simulink library "GFL_Lib"  (R2019b)
settings: Solver=VariableStepAuto  StartTime=0.0  StopTime=10.0  RelTol=1e-3
undefined symbols (not defined in the file or in its folder): Carm, Diff_CC_ki, Diff_CC_kp, fb, Ib2, Idcb, Ki_i, Ki_Wdiff_pu, Ki_Wtot_pu, Kp_i, Kp_Rvi_pu, Kp_Wdiff_pu, Kp_Wtot_pu, Lb, Lc_eq, Lc_pu, Lf_pu, Sb, Solver_Time_Step, Time_Step, Va0, Vb0, Vb1, Vb2, Vc0, Vdcb, Vm0, Vm0_d, Vm0_q, VSC01_id0, Vvsc0, wb, Zb
libraries: powerlib x90, Control_Lib x57, spsCurrentMeasurementLib x7, simulink x7, spsControlledCurrentSourceLib x6, $bdroot x5, Source_Lib x2, eeGeneralControl x2, powerlib_meascontrol x2, GFo_Lib x1
(part 3 of 5)

== system GFL_Lib/GFM_VC MMC/Bridge_Model ==
  vv_ref : Inport
  vdiff_ref : Inport  Port=2
  Bus1 : powerlib/Measurements/Three-Phase V-I Measurement  VoltageMeasurement=phase-to-ground  SetLabelV=off  LabelV=Vabc  Vpu=off  VpuLL=off  CurrentMeasurement=no  SetLabelI=off  LabelI=Iabc  Ipu=off  Pbase=100e6  Vbase=500e3  OutputType=Complex  PhasorSimulation=off  PSBequivalent=0
  Current Measurement : spsCurrentMeasurementLib/Current Measurement  PhasorSimulation=off  OutputType=Complex  PSBequivalent=0
  Decoupling voltage : Subsystem
  MMC Average Model : Subsystem
  Memory1 : Memory  InitialCondition=Udcn
  Modulation Index Generation : Subsystem
  Mux : Mux  Inputs=2
  NOT1 : Logic  Operator=NOT  IconShape=distinctive  AllPortsSameDT=off  OutDataTypeStr=boolean
  Step : Step  Time=Output_Delay  SampleTime=0
  Three-Phase Breaker1 : powerlib/Elements/Three-Phase Breaker  InitialState=closed  SwitchA=on  SwitchB=on  SwitchC=on  SwitchTimes="[4/60  10/60]"  External=on  BreakerResistance=1e-5*Zb  SnubberResistance=1e6  SnubberCapacitance=inf  Measurements=None
  Three-Phase Breaker2 : powerlib/Elements/Three-Phase Breaker  InitialState=open  SwitchA=on  SwitchB=on  SwitchC=on  SwitchTimes="[4/60  10/60]"  External=on  BreakerResistance=1e-5*Zb  SnubberResistance=1e6  SnubberCapacitance=inf  Measurements=None
  Three-Phase Source : powerlib/Electrical Sources/Three-Phase Source  InternalConnection=Yg  VoltagePhases=off  Voltage=Vm0*Un1  PhaseAngle=Theta_Vm0  Voltage_phases=[25e3 25e3 25e3]/sqrt(3)  PhaseAngles_phases=[0 -120 +120]  Frequency=fb  NonIdealSource=on  SpecifyImpedance=off  Resistance=Rarm_pu/2*Zb  Inductance=Larm_pu/2*Lb  ShortCircuitLevel=100e6  BaseVoltage=Un1  XRratio=7  BusType=swing  Pref=0.3  Qref=0  Prefabc=[10e3, 10e3, 10e3]  Qrefabc=[0, 0, 0]  Qmin=-Inf  Qmax=Inf
  Voltage Measurement : powerlib/Measurements/Voltage Measurement  PhasorSimulation=off  OutputType=Complex  PSBequivalent=0
  PhA : PMIOPort  Side=Right
  PhB : PMIOPort  Port=2  Side=Right
  PhC : PMIOPort  Port=3  Side=Right
  Vdc+ : PMIOPort  Port=4  Side=Left
  Vdc- : PMIOPort  Port=5  Side=Left
  m_dc : Outport
  m : Outport  Port=2
  vv : Outport  Port=3
  wires:
  NOT1/1 -> Three-Phase Breaker1/1
  Step/1 -> Three-Phase Breaker2/1, NOT1/1
  vv_ref/1 -> Decoupling voltage/1(Vv_ref)
  vdiff_ref/1 -> Decoupling voltage/2(Vdiff_ref)
  Decoupling voltage/1(Vmu_ref) -> Modulation Index Generation/1(vmu_ref)
  Decoupling voltage/2(Vml_ref) -> Modulation Index Generation/2(vml_ref)
  MMC Average Model/1(m) -> m/1
  Voltage Measurement/1 -> Memory1/1  "Vdc"
  Current Measurement/1 -> Mux/2  "Idc"
  Mux/1 -> m_dc/1
  Modulation Index Generation/1(mul) -> MMC Average Model/1(mul)
  Bus1/1 -> vv/1
  Memory1/1 -> Mux/1
  connections:
  Three-Phase Breaker1/LConn1 -- Bus1/LConn1 -- Three-Phase Breaker2/LConn1
  Three-Phase Breaker1/LConn2 -- Bus1/LConn2 -- Three-Phase Breaker2/LConn2
  Three-Phase Breaker1/LConn3 -- Bus1/LConn3 -- Three-Phase Breaker2/LConn3
  MMC Average Model/LConn1 -- Three-Phase Breaker2/RConn1
  MMC Average Model/LConn2 -- Three-Phase Breaker2/RConn2
  MMC Average Model/LConn3 -- Three-Phase Breaker2/RConn3
  Three-Phase Source/RConn1 -- Three-Phase Breaker1/RConn1
  Three-Phase Source/RConn2 -- Three-Phase Breaker1/RConn2
  Three-Phase Source/RConn3 -- Three-Phase Breaker1/RConn3
  MMC Average Model/RConn1 -- Current Measurement/RConn1 -- Voltage Measurement/LConn1
  MMC Average Model/RConn2 -- Voltage Measurement/LConn2 -- Vdc-/RConn1
  Current Measurement/LConn1 -- Vdc+/RConn1
  PhB/RConn1 -- Bus1/RConn2
  PhC/RConn1 -- Bus1/RConn3
  PhA/RConn1 -- Bus1/RConn1

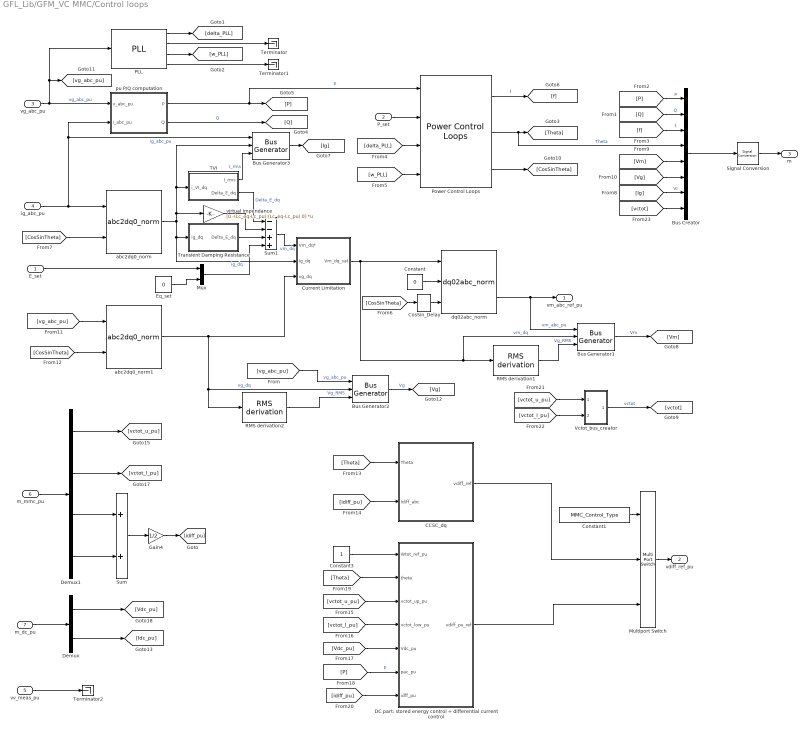
== system GFL_Lib/GFM_VC MMC/Control loops ==
  E_set : Inport
  P_set : Inport  Port=2
  vg_abc_pu : Inport  Port=3
  ig_abc_pu : Inport  Port=4
  vv_meas_pu : Inport  Port=5
  m_mmc_pu : Inport  Port=6
  m_dc_pu : Inport  Port=7
  " pu P/Q computation" : Subsystem  DialogController=POWERSYS.PowerSysDialog
  Bus Creator : BusCreator  Inputs=8
  Bus Generator1 : Control_Lib/Bus Generator  Gpu=Vb1
      settings: SourceProductName=VSC4SPS
  Bus Generator2 : Control_Lib/Bus Generator  Gpu=Vb1
      settings: SourceProductName=VSC4SPS
  Bus Generator3 : Control_Lib/Bus Generator  Gpu=Vb1
      settings: SourceProductName=VSC4SPS
  CCSC_dq : Subsystem
  Constant : Constant  Value=0
  Constant1 : Constant  Value=MMC_Control_Type
  Constant3 : Constant
  CosSin_Delay : Control_Lib/CosSin_Delay  dTheta=wb*Output_Delay
      settings: SourceProductName=VSC4SPS
  Current Limitation : Subsystem
  DC part: stored energy control + differential current control : Subsystem
  Demux : Demux  Outputs=2
  Demux1 : Demux  Outputs=[3 3 3 3]
  Eq_set : Constant  Value=0
  Gain4 : Gain  Gain=1/2
  Multiport Switch : MultiPortSwitch  Inputs=2
  Mux : Mux  Inputs=2
  PLL : Control_Lib/PLL  fb=fb  wn_PLL=wn_PLL  zeta_PLL=zeta_PLL  Theta0=Theta0
      settings: SourceProductName=VSC4SPS
  Power Control Loops : Control_Lib/Power Control Loops  Theta0_VSC=Theta_Vvsc0
      settings: SourceProductName=VSC4SPS
  RMS derivation1 : Control_Lib/RMS derivation  SystemSampleTime=-1  Latency=0  AutoFrameSizeCalculation=off
      settings: SourceProductName=VSC4SPS
  RMS derivation2 : Control_Lib/RMS derivation  SystemSampleTime=-1  Latency=0  AutoFrameSizeCalculation=off
      settings: SourceProductName=VSC4SPS
  Signal Conversion : SignalConversion  OverrideOpt=off
  Sum : Sum
  Sum1 : Sum  Inputs=--++
  TVI : Subsystem
  Terminator : Terminator
  Terminator1 : Terminator
  Terminator2 : Terminator
  Transient Damping Resistance : Subsystem
  Vctot_bus_creator : Subsystem
  abc2dq0_norm : Control_Lib/abc2dq0_norm  referenceAxisMode=Reference axis at 90 degrees behind phase_a  baseUpdateGain=1/sqrt(3)
      settings: SourceProductName=VSC4SPS
  abc2dq0_norm1 : Control_Lib/abc2dq0_norm  referenceAxisMode=Reference axis at 90 degrees behind phase_a  baseUpdateGain=1/sqrt(3)
      settings: SourceProductName=VSC4SPS
  dq02abc_norm : Control_Lib/dq02abc_norm  referenceAxisMode=Reference axis at 90 degrees behind phase_a  baseUpdateGain=sqrt(3)
      settings: SourceProductName=VSC4SPS
  virtual impendance : Gain  Gain=[0 -(Lc_eq-Lc_pu);(Lc_eq-Lc_pu) 0]  Multiplication=Matrix(K*u)
  vm_abc_ref_pu : Outport  VectorParamsAs1DForOutWhenUnconnected=off
  vdiff_ref_pu : Outport  Port=2
  m : Outport  Port=3  VectorParamsAs1DForOutWhenUnconnected=off
  wires:
  vv_meas_pu/1 -> Terminator2/1
  [vctot] -> Bus Creator/8
  [vctot_l_pu] -> Vctot_bus_creator/2(In2)
  Vctot_bus_creator/1(Out1) -> [vctot]  "vctot"
  [vctot_u_pu] -> Vctot_bus_creator/1(In1)
  Multiport Switch/1 -> vdiff_ref_pu/1
  PLL/4 -> Terminator1/1
  PLL/2 -> Terminator/1
  PLL/1 -> [delta_PLL]
  Constant/1 -> dq02abc_norm/2
  Power Control Loops/3 -> [CosSinTheta]
  PLL/3 -> [w_PLL]
  [Vg] -> Bus Creator/6
  Bus Creator/1 -> Signal Conversion/1
  [Ig] -> Bus Creator/7  "VI"
  [Vm] -> Bus Creator/5
  Eq_set/1 -> Mux/2
  Mux/1 -> Sum1/4
  TVI/1(I_rms) -> Bus Generator3/3  "I_rms"
  Transient Damping Resistance/1("Delta_E_dq ") -> Sum1/3
  TVI/2(Delta_E_dq) -> Sum1/1  "Delta_E_dq"
  [CosSinTheta] -> abc2dq0_norm/2
  [CosSinTheta] -> CosSin_Delay/1
  Power Control Loops/2 -> Bus Creator/4, [Theta]  "Theta"
  abc2dq0_norm/2 -> Transient Damping Resistance/1(ig_dq), Current Limitation/2(Ig_dq), Bus Generator3/2, TVI/1(i_VI_dq), virtual impendance/1  "ig_dq"
  ig_abc_pu/1 -> abc2dq0_norm/1, Bus Generator3/1, " pu P/Q computation"/2(i_abc_pu)  "ig_abc_pu"
  " pu P/Q computation"/1(P) -> Power Control Loops/1, [P]  "P"
  vg_abc_pu/1 -> PLL/1, [vg_abc_pu], " pu P/Q computation"/1(v_abc_pu)  "vg_abc_pu"
  Power Control Loops/1 -> [f]  "f"
  P_set/1 -> Power Control Loops/2
  [delta_PLL] -> Power Control Loops/3
  Current Limitation/1(Vm_dq_sat) -> Bus Generator1/2, RMS derivation1/1, dq02abc_norm/1  "vm_dq"
  " pu P/Q computation"/2(Q) -> [Q]  "Q"
  E_set/1 -> Mux/1
  dq02abc_norm/2 -> Bus Generator1/1, vm_abc_ref_pu/1  "vm_abc_pu"
  [f] -> Bus Creator/3  "f"
  [Q] -> Bus Creator/2  "Q"
  [P] -> Bus Creator/1  "P"
  Signal Conversion/1 -> m/1
  Sum1/1 -> Current Limitation/1(Vm_dq*)  "vm_dq"
  [vg_abc_pu] -> abc2dq0_norm1/1
  [CosSinTheta] -> abc2dq0_norm1/2
  Demux1/2 -> [vctot_l_pu]
  Demux1/1 -> [vctot_u_pu]
  m_mmc_pu/1 -> Demux1/1
  Demux/2 -> [Idc_pu]
  Demux/1 -> [Vdc_pu]
  m_dc_pu/1 -> Demux/1
  Gain4/1 -> [idiff_pu]
  Sum/1 -> Gain4/1
  Demux1/3 -> Sum/1
  Demux1/4 -> Sum/2
  [vctot_u_pu] -> DC part: stored energy control + differential current control/3(vctot_up_pu)
  [vctot_l_pu] -> DC part: stored energy control + differential current control/4(vctot_low_pu)
  [Vdc_pu] -> DC part: stored energy control + differential current control/5(Vdc_pu)
  [P] -> DC part: stored energy control + differential current control/6(pac_pu)  "P"
  Constant3/1 -> DC part: stored energy control + differential current control/1(Wtot_ref_pu)
  [Theta] -> DC part: stored energy control + differential current control/2(theta)
  [idiff_pu] -> DC part: stored energy control + differential current control/7(idff_pu)
  [w_PLL] -> Power Control Loops/4
  CosSin_Delay/1 -> dq02abc_norm/3
  [Theta] -> CCSC_dq/1(Theta)
  CCSC_dq/1(vdiff_ref) -> Multiport Switch/2
  [idiff_pu] -> CCSC_dq/2(Idiff_abc)
  virtual impendance/1 -> Sum1/2
  DC part: stored energy control + differential current control/1(vdiff_pu_ref) -> Multiport Switch/3
  Constant1/1 -> Multiport Switch/1
  Bus Generator1/1 -> [Vm]  "Vm"
  RMS derivation1/1 -> Bus Generator1/3  "Vg_RMS"
  RMS derivation2/1 -> Bus Generator2/3  "Vg_RMS"
  Bus Generator2/1 -> [Vg]  "Vg"
  [vg_abc_pu] -> Bus Generator2/1  "vg_abc_pu"
  abc2dq0_norm1/2 -> RMS derivation2/1, Bus Generator2/2, Current Limitation/3(vg_dq)  "vg_dq"
  Bus Generator3/1 -> [Ig]

== system GFL_Lib/GFM_VC MMC/Normalization_dc ==
  m_dc : Inport
  Demux : Demux  Outputs=2
  Gain11 : Gain  Gain=1/Vdcb
  Gain12 : Gain  Gain=1/Idcb
  Mux : Mux  Inputs=2
  m_dc_pu : Outport
  wires:
  Mux/1 -> m_dc_pu/1
  Demux/2 -> Gain12/1
  Gain12/1 -> Mux/2  "Idc_pu"
  Gain11/1 -> Mux/1  "Vdc_pu"
  Demux/1 -> Gain11/1
  m_dc/1 -> Demux/1

== system GFL_Lib/GFM_VC MMC/Normalizaton ==
  m_mmc : Inport
  Demux : Demux  Outputs=[3 3 3 3]
  Gain : Gain  Gain=1/Idcb
  Gain3 : Gain  Gain=1/Idcb
  Gain6 : Gain  Gain=1/Vdcb
  Gain8 : Gain  Gain=1/Vdcb
  Mux : Mux
  m_mmc_pu : Outport
  wires:
  m_mmc/1 -> Demux/1
  Mux/1 -> m_mmc_pu/1
  Demux/3 -> Gain/1
  Gain/1 -> Mux/3  "i_arm_u_pu"
  Demux/4 -> Gain3/1
  Gain3/1 -> Mux/4  "i_arm_l_pu"
  Demux/2 -> Gain8/1
  Gain6/1 -> Mux/1  "vctot_u_pu"
  Demux/1 -> Gain6/1
  Gain8/1 -> Mux/2  "vctot_l_pu"

== system GFL_Lib/Mean Model 2-Level L-filter with DC Link/Bridge_Model ==
  Uref : Inport
  Constant : Constant
  Memory1 : Memory
  NOT1 : Logic  Operator=NOT  IconShape=distinctive  AllPortsSameDT=off  OutDataTypeStr=boolean
  Saturation : Saturate  UpperLimit=1  LowerLimit=-1
  Terminator : Terminator
  Three-Phase Breaker2 : powerlib/Elements/Three-Phase Breaker  InitialState=open  SwitchA=on  SwitchB=on  SwitchC=on  SwitchTimes="[4/60  10/60]"  External=on  BreakerResistance=1e-5*Zb  SnubberResistance=1e6  SnubberCapacitance=inf  Measurements=None
  Three-Phase Breaker3 : powerlib/Elements/Three-Phase Breaker  InitialState=closed  SwitchA=on  SwitchB=on  SwitchC=on  SwitchTimes="[4/60  10/60]"  External=on  BreakerResistance=1e-5*Zb  SnubberResistance=1e6  SnubberCapacitance=inf  Measurements=None
  Three-Phase Source : powerlib/Electrical Sources/Three-Phase Source  InternalConnection=Yg  VoltagePhases=off  Voltage=Vvsc0*Un1  PhaseAngle=Theta_vsc0  Voltage_phases=[25e3 25e3 25e3]/sqrt(3)  PhaseAngles_phases=[0 -120 +120]  Frequency=fb  NonIdealSource=off  SpecifyImpedance=off  Resistance=0  Inductance=0  ShortCircuitLevel=100e6  BaseVoltage=VSC01_Un1  XRratio=7  BusType=swing  Pref=0.3  Qref=0  Prefabc=[10e3, 10e3, 10e3]  Qrefabc=[0, 0, 0]  Qmin=-Inf  Qmax=Inf
  Universal Bridge : powerlib/Power Electronics/Universal Bridge  Arms=3  SnubberResistance=1e5  SnubberCapacitance=inf  Device=Average-model based VSC  Ron=1e-3  Lon=0  ForwardVoltages="[  0  0  ]"  ForwardVoltage=0  GTOparameters=[ 10e-6 , 20e-6 ]  IGBTparameters=[ 1e-6 , 2e-6 ]  Measurements=None  Measurements_2=None  converterType=Rectifier
  Vdc : powerlib/Measurements/Voltage Measurement  PhasorSimulation=off  OutputType=Complex  PSBequivalent=0
  mp3 : Gain  Gain=2/Udcn
  PhA : PMIOPort  Side=Right
  PhB : PMIOPort  Port=2  Side=Right
  PhC : PMIOPort  Port=3  Side=Right
  Vdc+ : PMIOPort  Port=4  Side=Left
  Vdc- : PMIOPort  Port=5  Side=Left
  wires:
  Vdc/1 -> Terminator/1
  Uref/1 -> mp3/1
  mp3/1 -> Saturation/1
  Constant/1 -> Memory1/1
  NOT1/1 -> Three-Phase Breaker3/1
  Saturation/1 -> Universal Bridge/1
  Memory1/1 -> Three-Phase Breaker2/1, NOT1/1
  connections:
  Vdc-/RConn1 -- Universal Bridge/RConn2 -- Vdc/LConn2
  Vdc+/RConn1 -- Universal Bridge/RConn1 -- Vdc/LConn1
  PhC/RConn1 -- Three-Phase Breaker3/LConn3 -- Three-Phase Breaker2/LConn3
  PhB/RConn1 -- Three-Phase Breaker3/LConn2 -- Three-Phase Breaker2/LConn2
  PhA/RConn1 -- Three-Phase Breaker3/LConn1 -- Three-Phase Breaker2/LConn1
  Three-Phase Breaker2/RConn3 -- Universal Bridge/LConn3
  Three-Phase Breaker2/RConn2 -- Universal Bridge/LConn2
  Three-Phase Breaker2/RConn1 -- Universal Bridge/LConn1
  Three-Phase Breaker3/RConn1 -- Three-Phase Source/RConn1
  Three-Phase Breaker3/RConn2 -- Three-Phase Source/RConn2
  Three-Phase Breaker3/RConn3 -- Three-Phase Source/RConn3

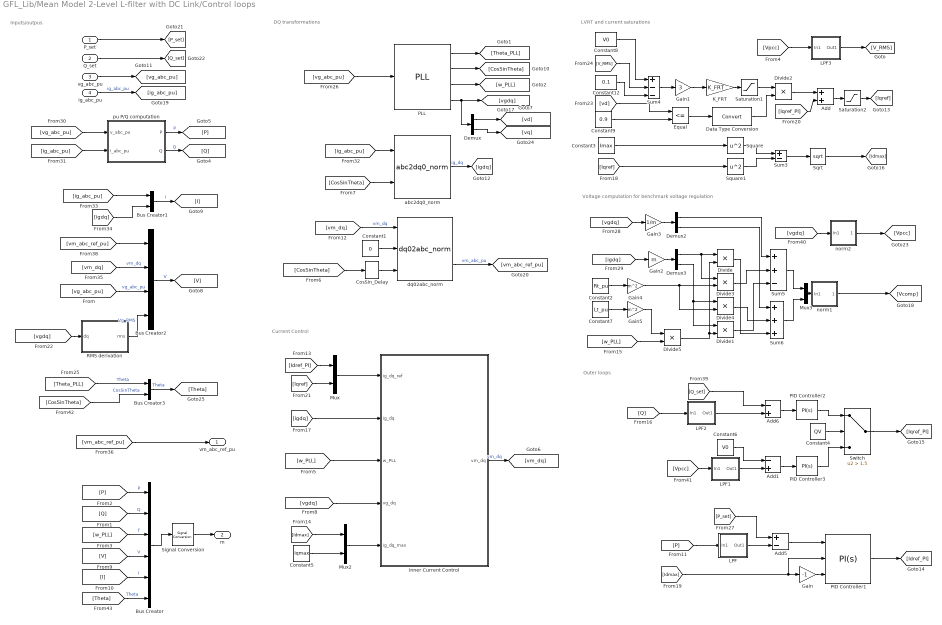
== system GFL_Lib/Mean Model 2-Level L-filter with DC Link/Control loops ==
  note: Voltage computation for benchmark voltage regulation
  note: LVRT and current saturations
  note: Outer loops
  note: Current Control
  note: DQ transformations
  note: Inputs/outpus
  P_set : Inport
  Q_set : Inport  Port=2
  vg_abc_pu : Inport  Port=3
  ig_abc_pu : Inport  Port=4
  " pu P/Q computation" : Subsystem  DialogController=POWERSYS.PowerSysDialog
  Add : Sum
  Add1 : Sum  Inputs=-+
  Add5 : Sum  Inputs=+-
  Add6 : Sum  Inputs=-+
  Bus Creator : BusCreator  Inputs=6
  Bus Creator1 : BusCreator  Inputs=2
  Bus Creator2 : BusCreator  Inputs=4
  Bus Creator3 : BusCreator  Inputs=2
  Constant1 : Constant  Value=0
  Constant12 : Constant  Value=0.1
  Constant2 : Constant  Value=Rt_pu
  Constant3 : Constant  Value=Imax
  Constant4 : Constant  Value=QV
  Constant5 : Constant  Value=Iqmax
  Constant6 : Constant  Value=V0
  Constant7 : Constant  Value=Lt_pu
  Constant8 : Constant  Value=V0
  Constant9 : Constant  Value=0.9
  CosSin_Delay : Control_Lib/CosSin_Delay  dTheta=wb*Solver_Time_Step
      settings: SourceProductName=VSC4SPS
  Data Type Conversion : DataTypeConversion
  Demux : Demux  Outputs=[1 1]
  Demux2 : Demux  Outputs=2
  Demux3 : Demux  Outputs=2
  Divide{,1..5} (6 alike) : Product  Inputs=**
  Equal : RelationalOperator  Operator=<=  OutDataTypeStr=boolean  RndMeth=Simplest
  Gain : Gain  Gain=-1
  Gain1 : Gain  Gain=3
  Gain2 : Gain  Gain=m
  Gain3 : Gain  Gain=1/m
  Gain4 : Gain  Gain=m^2
  Gain5 : Gain  Gain=m^2
  Inner Current Control : Subsystem
  K_FRT : Gain  Gain=K_FRT
  LPF : Subsystem
  LPF1 : Subsystem
  LPF2 : Subsystem
  LPF3 : Subsystem
  Mux : Mux  Inputs=2
  Mux2 : Mux  Inputs=2
  Mux3 : Mux  Inputs=2
  PID Controller1 : simulink/Continuous/PID Controller  Controller=PI  Form=Parallel  TimeDomain=Continuous-time  SampleTime=-1  IntegratorMethod=Forward Euler  FilterMethod=Forward Euler  ControllerParametersSource=internal  P=w_P/w_LPF  I=w_P  D=0  UseFilter=on  N=100  TunerSelectOption=Transfer Function Based (PID Tuner App)  InitialConditionSource=internal  InitialConditionForIntegrator=P0/V0  InitialConditionForFilter=0  DifferentiatorICPrevScaledInput=0  ExternalReset=none  TrackingMode=off  Kt=1  LimitOutput=on  UpperSaturationLimit=inf  LowerSaturationLimit=-inf  LinearizeAsGain=on  AntiWindupMode=clamping  Kb=1  POutMin=[]  POutMax=[]  IOutMin=[]  IOutMax=[]  DOutMin=[]  DOutMax=[]  NOutMin=[]  NOutMax=[]  SumOutMin=[]  SumOutMax=[]  SaturationOutMin=[]  SaturationOutMax=[]  PParamMin=[]  PParamMax=[]  IParamMin=[]  IParamMax=[]  DParamMin=[]  DParamMax=[]  NParamMin=[]  NParamMax=[]  KbParamMin=[]  KbParamMax=[]  KtParamMin=[]  KtParamMax=[]  KbOutMin=[]  KbOutMax=[]  KtOutMin=[]  KtOutMax=[]  IntegratorOutMin=[]  IntegratorOutMax=[]  FilterOutMin=[]  FilterOutMax=[]  SumI1OutMin=[]  SumI1OutMax=[]  SumI2OutMin=[]  SumI2OutMax=[]  SumI3OutMin=[]  SumI3OutMax=[]  SumI4OutMin=[]  SumI4OutMax=[]  SumDOutMin=[]  SumDOutMax=[]  DifferentiatorOutMin=[]  DifferentiatorOutMax=[]  FilterDiffOutCoefMin=[]  FilterDiffOutCoefMax=[]  ReciprocalOutMin=[]  ReciprocalOutMax=[]  SumDenOutMin=[]  SumDenOutMax=[]  SumNumOutMin=[]  SumNumOutMax=[]  DivideOutMin=[]  DivideOutMax=[]  IntegratorContinuousStateAttributes=''  IntegratorStateMustResolveToSignalObject=off  IntegratorRTWStateStorageClass=Auto  FilterContinuousStateAttributes=''  FilterStateMustResolveToSignalObject=off  FilterRTWStateStorageClass=Auto  ParallelPVariant=InternalParameters  IdealPVariant=Disabled  IVariant=InternalParameters  DVariant=Disabled  IntegratorVariant=Continuous  SatVariant=External  AWVariant=ContClampingParallel  PCopyVariant=Disabled  TRVariant=Disabled  FdbkBlocksVariant=Forward  IdealPFdbkVariant=Disabled  SatFdbkVariant=Disabled  DerivativeFilterVariant=Disabled  NVariant=Disabled  NCopyVariant=Disabled_SignalSpec  FilterICVariant=Disabled  IntegratorICVariant=InternalICs  ExternalResetVariant=Disabled  TRSumVariant=Passthrough  SumFdbkVariant=Disabled  SumVariant=Sum_PI
  PID Controller2 : simulink/Continuous/PID Controller  Controller=PI  Form=Parallel  TimeDomain=Continuous-time  SampleTime=-1  IntegratorMethod=Forward Euler  FilterMethod=Forward Euler  ControllerParametersSource=internal  P=w_P/w_LPF  I=w_P  D=0  UseFilter=on  N=100  TunerSelectOption=Transfer Function Based (PID Tuner App)  InitialConditionSource=internal  InitialConditionForIntegrator=-Q0/V0  InitialConditionForFilter=0  DifferentiatorICPrevScaledInput=0  ExternalReset=none  TrackingMode=off  Kt=1  LimitOutput=on  UpperSaturationLimit=Iqmax  LowerSaturationLimit=-Iqmax  LinearizeAsGain=on  AntiWindupMode=clamping  Kb=1  POutMin=[]  POutMax=[]  IOutMin=[]  IOutMax=[]  DOutMin=[]  DOutMax=[]  NOutMin=[]  NOutMax=[]  SumOutMin=[]  SumOutMax=[]  SaturationOutMin=[]  SaturationOutMax=[]  PParamMin=[]  PParamMax=[]  IParamMin=[]  IParamMax=[]  DParamMin=[]  DParamMax=[]  NParamMin=[]  NParamMax=[]  KbParamMin=[]  KbParamMax=[]  KtParamMin=[]  KtParamMax=[]  KbOutMin=[]  KbOutMax=[]  KtOutMin=[]  KtOutMax=[]  IntegratorOutMin=[]  IntegratorOutMax=[]  FilterOutMin=[]  FilterOutMax=[]  SumI1OutMin=[]  SumI1OutMax=[]  SumI2OutMin=[]  SumI2OutMax=[]  SumI3OutMin=[]  SumI3OutMax=[]  SumI4OutMin=[]  SumI4OutMax=[]  SumDOutMin=[]  SumDOutMax=[]  DifferentiatorOutMin=[]  DifferentiatorOutMax=[]  FilterDiffOutCoefMin=[]  FilterDiffOutCoefMax=[]  ReciprocalOutMin=[]  ReciprocalOutMax=[]  SumDenOutMin=[]  SumDenOutMax=[]  SumNumOutMin=[]  SumNumOutMax=[]  DivideOutMin=[]  DivideOutMax=[]  IntegratorContinuousStateAttributes=''  IntegratorStateMustResolveToSignalObject=off  IntegratorRTWStateStorageClass=Auto  FilterContinuousStateAttributes=''  FilterStateMustResolveToSignalObject=off  FilterRTWStateStorageClass=Auto  ParallelPVariant=InternalParameters  IdealPVariant=Disabled  IVariant=InternalParameters  DVariant=Disabled  IntegratorVariant=Continuous  SatVariant=Enabled  AWVariant=ContClampingParallel  PCopyVariant=Disabled  TRVariant=Disabled  FdbkBlocksVariant=Forward  IdealPFdbkVariant=Disabled  SatFdbkVariant=Disabled  DerivativeFilterVariant=Disabled  NVariant=Disabled  NCopyVariant=Disabled_SignalSpec  FilterICVariant=Disabled  IntegratorICVariant=InternalICs  ExternalResetVariant=Disabled  TRSumVariant=Passthrough  SumFdbkVariant=Disabled  SumVariant=Sum_PI
  PID Controller3 : simulink/Continuous/PID Controller  Controller=PI  Form=Parallel  TimeDomain=Continuous-time  SampleTime=-1  IntegratorMethod=Forward Euler  FilterMethod=Forward Euler  ControllerParametersSource=internal  P=w_V/w_LPF  I=w_V  D=0  UseFilter=on  N=100  TunerSelectOption=Transfer Function Based (PID Tuner App)  InitialConditionSource=internal  InitialConditionForIntegrator=-Q0/V0  InitialConditionForFilter=0  DifferentiatorICPrevScaledInput=0  ExternalReset=none  TrackingMode=off  Kt=1  LimitOutput=on  UpperSaturationLimit=Iqmax  LowerSaturationLimit=-Iqmax  LinearizeAsGain=on  AntiWindupMode=clamping  Kb=1  POutMin=[]  POutMax=[]  IOutMin=[]  IOutMax=[]  DOutMin=[]  DOutMax=[]  NOutMin=[]  NOutMax=[]  SumOutMin=[]  SumOutMax=[]  SaturationOutMin=[]  SaturationOutMax=[]  PParamMin=[]  PParamMax=[]  IParamMin=[]  IParamMax=[]  DParamMin=[]  DParamMax=[]  NParamMin=[]  NParamMax=[]  KbParamMin=[]  KbParamMax=[]  KtParamMin=[]  KtParamMax=[]  KbOutMin=[]  KbOutMax=[]  KtOutMin=[]  KtOutMax=[]  IntegratorOutMin=[]  IntegratorOutMax=[]  FilterOutMin=[]  FilterOutMax=[]  SumI1OutMin=[]  SumI1OutMax=[]  SumI2OutMin=[]  SumI2OutMax=[]  SumI3OutMin=[]  SumI3OutMax=[]  SumI4OutMin=[]  SumI4OutMax=[]  SumDOutMin=[]  SumDOutMax=[]  DifferentiatorOutMin=[]  DifferentiatorOutMax=[]  FilterDiffOutCoefMin=[]  FilterDiffOutCoefMax=[]  ReciprocalOutMin=[]  ReciprocalOutMax=[]  SumDenOutMin=[]  SumDenOutMax=[]  SumNumOutMin=[]  SumNumOutMax=[]  DivideOutMin=[]  DivideOutMax=[]  IntegratorContinuousStateAttributes=''  IntegratorStateMustResolveToSignalObject=off  IntegratorRTWStateStorageClass=Auto  FilterContinuousStateAttributes=''  FilterStateMustResolveToSignalObject=off  FilterRTWStateStorageClass=Auto  ParallelPVariant=InternalParameters  IdealPVariant=Disabled  IVariant=InternalParameters  DVariant=Disabled  IntegratorVariant=Continuous  SatVariant=Enabled  AWVariant=ContClampingParallel  PCopyVariant=Disabled  TRVariant=Disabled  FdbkBlocksVariant=Forward  IdealPFdbkVariant=Disabled  SatFdbkVariant=Disabled  DerivativeFilterVariant=Disabled  NVariant=Disabled  NCopyVariant=Disabled_SignalSpec  FilterICVariant=Disabled  IntegratorICVariant=InternalICs  ExternalResetVariant=Disabled  TRSumVariant=Passthrough  SumFdbkVariant=Disabled  SumVariant=Sum_PI
  PLL : Control_Lib/PLL  fb=fb  wn_PLL=500  zeta_PLL=1  Theta0=Theta0
      settings: SourceProductName=VSC4SPS
  RMS derivation : Subsystem
  Saturation1 : Saturate  UpperLimit=Imax  LowerLimit=-Imax
  Saturation2 : Saturate  UpperLimit=Imax  LowerLimit=-Imax
  Signal Conversion : SignalConversion  OverrideOpt=off
  Sqrt : Sqrt  SaturateOnIntegerOverflow=on
  Square : Math  Operator=square  SaturateOnIntegerOverflow=on
  Square1 : Math  Operator=square  SaturateOnIntegerOverflow=on
  Sum3 : Sum  Inputs=+-
  Sum4 : Sum  Inputs=+--
  Sum5 : Sum  Inputs=++-
  Sum6 : Sum  Inputs=+++
  Switch : Switch  Criteria=u2 > Threshold  Threshold=1.5
  abc2dq0_norm : Control_Lib/abc2dq0_norm  referenceAxisMode=Reference axis at 90 degrees behind phase_a  baseUpdateGain=1/sqrt(3)
      settings: SourceProductName=VSC4SPS
  dq02abc_norm : Control_Lib/dq02abc_norm  referenceAxisMode=Reference axis at 90 degrees behind phase_a  baseUpdateGain=sqrt(3)
      settings: SourceProductName=VSC4SPS
  norm1 : Subsystem
  norm2 : Subsystem
  vm_abc_ref_pu : Outport  VectorParamsAs1DForOutWhenUnconnected=off
  m : Outport  Port=2  VectorParamsAs1DForOutWhenUnconnected=off
  wires:
  [vg_abc_pu] -> Bus Creator2/3  "vg_abc_pu"
  Constant1/1 -> dq02abc_norm/2
  Mux/1 -> Inner Current Control/1(ig_dq_ref)
  Signal Conversion/1 -> m/1
  [P] -> Bus Creator/1  "P"
  [Q] -> Bus Creator/2  "Q"
  [w_PLL] -> Bus Creator/3  "f"
  dq02abc_norm/2 -> [vm_abc_ref_pu]  "vm_abc_pu"
  " pu P/Q computation"/2(Q) -> [Q]  "Q"
  [vm_dq] -> dq02abc_norm/1  "vm_dq"
  [w_PLL] -> Inner Current Control/3(w_PLL)
  Inner Current Control/1(vm_dq) -> [vm_dq]  "vm_dq"
  vg_abc_pu/1 -> [vg_abc_pu]
  " pu P/Q computation"/1(P) -> [P]  "P"
  ig_abc_pu/1 -> [ig_abc_pu]  "ig_abc_pu"
  abc2dq0_norm/2 -> [igdq]  "ig_dq"
  [CosSinTheta] -> CosSin_Delay/1
  [CosSinTheta] -> abc2dq0_norm/2
  Bus Creator2/1 -> [V]  "V"
  [V] -> Bus Creator/4  "V"
  Bus Creator/1 -> Signal Conversion/1
  Bus Creator1/1 -> [I]  "I"
  [I] -> Bus Creator/5  "I"
  LPF2/1(Out1) -> Add6/2
  P_set/1 -> [P_set]
  Add6/1 -> PID Controller2/1
  [P] -> LPF/1(In1)
  Add5/1 -> PID Controller1/1
  [Iqref] -> Mux/2
  [Idref_PI] -> Mux/1
  [igdq] -> Inner Current Control/2(ig_dq)
  Saturation2/1 -> [Iqref]
  Sum4/1 -> Gain1/1
  [V_RMS] -> Sum4/2
  K_FRT/1 -> Saturation1/1
  Saturation1/1 -> Divide2/1
  Equal/1 -> Data Type Conversion/1
  Data Type Conversion/1 -> Divide2/2
  [vd] -> Equal/1
  Divide2/1 -> Add/1
  Constant12/1 -> Sum4/3
  Constant8/1 -> Sum4/1
  Constant9/1 -> Equal/2
  Constant4/1 -> Switch/2
  Add/1 -> Saturation2/1
  [Iqref_PI] -> Add/2
  Mux2/1 -> Inner Current Control/5(ig_dq_max)
  Constant5/1 -> Mux2/2
  [Idmax] -> Mux2/1
  [Q] -> LPF2/1(In1)
  Q_set/1 -> [Q_set]
  PID Controller2/1 -> Switch/1
  Add1/1 -> PID Controller3/1
  LPF1/1(Out1) -> Add1/2
  PID Controller3/1 -> Switch/3
  Square1/1 -> Sum3/2
  Sqrt/1 -> [Idmax]
  Sum3/1 -> Sqrt/1
  Constant3/1 -> Square/1
  Square/1 -> Sum3/1
  [Iqref] -> Square1/1
  Gain/1 -> PID Controller1/3
  [Idmax] -> PID Controller1/2, Gain/1
  Gain1/1 -> K_FRT/1
  Sum5/1 -> Mux3/1
  [vgdq] -> Gain3/1
  Demux2/2 -> Sum6/1
  Gain3/1 -> Demux2/1
  Constant2/1 -> Gain4/1
  norm1/1(Out1) -> [Vcomp]
  Divide1/1 -> Sum5/3
  Sum6/1 -> Mux3/2
  Mux3/1 -> norm1/1(In1)
  Divide/1 -> Sum6/3
  Divide5/1 -> Divide/2, Divide1/2
  Demux2/1 -> Sum5/1
  Divide3/1 -> Sum5/2
  Demux3/2 -> Divide1/1, Divide4/1
  Divide4/1 -> Sum6/2
  Demux3/1 -> Divide/1, Divide3/1
  PLL/1 -> [Theta_PLL]
  PLL/2 -> [CosSinTheta]
  PLL/3 -> [w_PLL]
  [w_PLL] -> Divide5/2
  Constant7/1 -> Gain5/1
  [Vpcc] -> LPF1/1(In1)
  Constant6/1 -> Add1/1
  [vg_abc_pu] -> PLL/1
  [vg_abc_pu] -> " pu P/Q computation"/1(v_abc_pu)
  [ig_abc_pu] -> " pu P/Q computation"/2(i_abc_pu)
  [ig_abc_pu] -> abc2dq0_norm/1
  [ig_abc_pu] -> Bus Creator1/1
  [igdq] -> Bus Creator1/2
  [vm_dq] -> Bus Creator2/2  "vm_dq"
  [vm_abc_ref_pu] -> vm_abc_ref_pu/1
  [vm_abc_ref_pu] -> Bus Creator2/1
  [vgdq] -> Inner Current Control/4(vg_dq)
  [P_set] -> Add5/1
  [Q_set] -> Add6/1
  [igdq] -> Gain2/1
  Gain2/1 -> Demux3/1
  Gain5/1 -> Divide5/1
  Gain4/1 -> Divide4/2, Divide3/2
  [vgdq] -> norm2/1(In1)
  norm2/1(Out1) -> [Vpcc]
  PLL/4 -> Demux/1, [vgdq]
  Demux/1 -> [vd]
  Demux/2 -> [vq]
  PID Controller1/1 -> [Idref_PI]
  Switch/1 -> [Iqref_PI]
  LPF/1(Out1) -> Add5/2
  [vgdq] -> RMS derivation/1(dq)
  RMS derivation/1(rms) -> Bus Creator2/4  "Vg_RMS"
  [Theta_PLL] -> Bus Creator3/1  "Theta"
  [CosSinTheta] -> Bus Creator3/2  "CosSinTheta"
  Bus Creator3/1 -> [Theta]  "Theta"
  [Theta] -> Bus Creator/6  "Theta"
  CosSin_Delay/1 -> dq02abc_norm/3
  LPF3/1(Out1) -> [V_RMS]
  [Vpcc] -> LPF3/1(In1)

== system GFL_Lib/Mean Model 2-Level L-filter_old/Bridge_Model ==
  Uref : Inport
  Constant : Constant
  Memory1 : Memory
  NOT1 : Logic  Operator=NOT  IconShape=distinctive  AllPortsSameDT=off  OutDataTypeStr=boolean
  Saturation : Saturate  UpperLimit=1  LowerLimit=-1
  Terminator : Terminator
  Three-Phase Breaker2 : powerlib/Elements/Three-Phase Breaker  InitialState=open  SwitchA=on  SwitchB=on  SwitchC=on  SwitchTimes="[4/60  10/60]"  External=on  BreakerResistance=1e-5*Zb  SnubberResistance=1e6  SnubberCapacitance=inf  Measurements=None
  Three-Phase Breaker3 : powerlib/Elements/Three-Phase Breaker  InitialState=closed  SwitchA=on  SwitchB=on  SwitchC=on  SwitchTimes="[4/60  10/60]"  External=on  BreakerResistance=1e-5*Zb  SnubberResistance=1e6  SnubberCapacitance=inf  Measurements=None
  Three-Phase Source : powerlib/Electrical Sources/Three-Phase Source  InternalConnection=Yg  VoltagePhases=off  Voltage=Vm0*Un1  PhaseAngle=Theta_Vm0  Voltage_phases=[25e3 25e3 25e3]/sqrt(3)  PhaseAngles_phases=[0 -120 +120]  Frequency=fb  NonIdealSource=off  SpecifyImpedance=off  Resistance=0  Inductance=0  ShortCircuitLevel=100e6  BaseVoltage=VSC01_Un1  XRratio=7  BusType=swing  Pref=0.3  Qref=0  Prefabc=[10e3, 10e3, 10e3]  Qrefabc=[0, 0, 0]  Qmin=-Inf  Qmax=Inf
  Universal Bridge : powerlib/Power Electronics/Universal Bridge  Arms=3  SnubberResistance=1e5  SnubberCapacitance=inf  Device=Average-model based VSC  Ron=1e-3  Lon=0  ForwardVoltages="[  0  0  ]"  ForwardVoltage=0  GTOparameters=[ 10e-6 , 20e-6 ]  IGBTparameters=[ 1e-6 , 2e-6 ]  Measurements=None  Measurements_2=None  converterType=Rectifier
  Vdc : powerlib/Measurements/Voltage Measurement  PhasorSimulation=off  OutputType=Complex  PSBequivalent=0
  mp3 : Gain  Gain=2/Udcn
  PhA : PMIOPort  Side=Right
  PhB : PMIOPort  Port=2  Side=Right
  PhC : PMIOPort  Port=3  Side=Right
  Vdc+ : PMIOPort  Port=4  Side=Left
  Vdc- : PMIOPort  Port=5  Side=Left
  wires:
  Vdc/1 -> Terminator/1
  Uref/1 -> mp3/1
  mp3/1 -> Saturation/1
  Constant/1 -> Memory1/1
  NOT1/1 -> Three-Phase Breaker3/1
  Saturation/1 -> Universal Bridge/1
  Memory1/1 -> Three-Phase Breaker2/1, NOT1/1
  connections:
  Vdc-/RConn1 -- Universal Bridge/RConn2 -- Vdc/LConn2
  Vdc+/RConn1 -- Universal Bridge/RConn1 -- Vdc/LConn1
  PhC/RConn1 -- Three-Phase Breaker3/LConn3 -- Three-Phase Breaker2/LConn3
  PhB/RConn1 -- Three-Phase Breaker3/LConn2 -- Three-Phase Breaker2/LConn2
  PhA/RConn1 -- Three-Phase Breaker3/LConn1 -- Three-Phase Breaker2/LConn1
  Three-Phase Breaker2/RConn3 -- Universal Bridge/LConn3
  Three-Phase Breaker2/RConn2 -- Universal Bridge/LConn2
  Three-Phase Breaker2/RConn1 -- Universal Bridge/LConn1
  Three-Phase Breaker3/RConn1 -- Three-Phase Source/RConn1
  Three-Phase Breaker3/RConn2 -- Three-Phase Source/RConn2
  Three-Phase Breaker3/RConn3 -- Three-Phase Source/RConn3

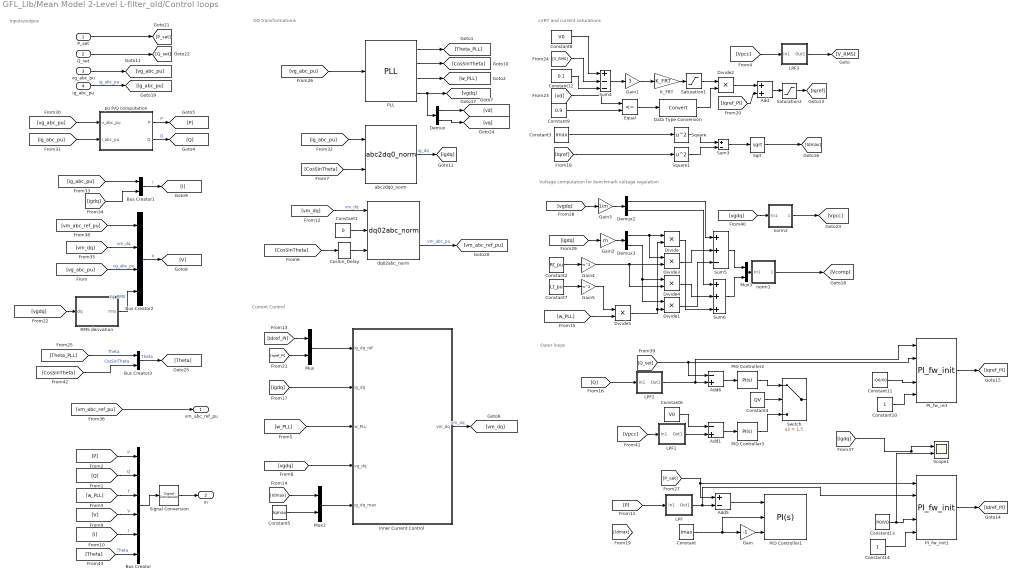
== system GFL_Lib/Mean Model 2-Level L-filter_old/Control loops ==
  note: Voltage computation for benchmark voltage regulation
  note: LVRT and current saturations
  note: Outer loops
  note: Current Control
  note: DQ transformations
  note: Inputs/outpus
  P_set : Inport
  Q_set : Inport  Port=2
  vg_abc_pu : Inport  Port=3
  ig_abc_pu : Inport  Port=4
  " pu P/Q computation" : Subsystem  DialogController=POWERSYS.PowerSysDialog
  Add : Sum
  Add1 : Sum  Inputs=-+
  Add5 : Sum  Inputs=+-
  Add6 : Sum  Inputs=-+
  Bus Creator : BusCreator  Inputs=6
  Bus Creator1 : BusCreator  Inputs=2
  Bus Creator2 : BusCreator  Inputs=4
  Bus Creator3 : BusCreator  Inputs=2
  Constant : Constant  Value=Imax
  Constant1 : Constant  Value=0
  Constant10 : Constant
  Constant11 : Constant  Value=-Q0/V0
  Constant12 : Constant  Value=0.1
  Constant13 : Constant  Value=P0/V0
  Constant14 : Constant
  Constant2 : Constant  Value=Rt_pu
  Constant3 : Constant  Value=Imax
  Constant4 : Constant  Value=QV
  Constant5 : Constant  Value=Iqmax
  Constant6 : Constant  Value=V0
  Constant7 : Constant  Value=Lt_pu
  Constant8 : Constant  Value=V0
  Constant9 : Constant  Value=0.9
  CosSin_Delay : Control_Lib/CosSin_Delay  dTheta=wb*Output_Delay
      settings: SourceProductName=VSC4SPS
  Data Type Conversion : DataTypeConversion
  Demux : Demux  Outputs=[1 1]
  Demux2 : Demux  Outputs=2
  Demux3 : Demux  Outputs=2
  Divide{,1..5} (6 alike) : Product  Inputs=**
  Equal : RelationalOperator  Operator=<=  OutDataTypeStr=boolean  RndMeth=Simplest
  Gain : Gain  Gain=-1
  Gain1 : Gain  Gain=3
  Gain2 : Gain  Gain=m
  Gain3 : Gain  Gain=1/m
  Gain4 : Gain  Gain=m^2
  Gain5 : Gain  Gain=m^2
  Inner Current Control : Subsystem
  K_FRT : Gain  Gain=K_FRT
  LPF : Subsystem
  LPF1 : Subsystem
  LPF2 : Subsystem
  LPF3 : Subsystem
  Mux : Mux  Inputs=2
  Mux2 : Mux  Inputs=2
  Mux3 : Mux  Inputs=2
  PID Controller1 : simulink/Continuous/PID Controller  Controller=PI  Form=Parallel  TimeDomain=Continuous-time  SampleTime=-1  IntegratorMethod=Forward Euler  FilterMethod=Forward Euler  ControllerParametersSource=internal  P=w_P/w_LPF  I=w_P  D=0  UseFilter=on  N=100  TunerSelectOption=Transfer Function Based (PID Tuner App)  InitialConditionSource=internal  InitialConditionForIntegrator=P0/V0  InitialConditionForFilter=0  DifferentiatorICPrevScaledInput=0  ExternalReset=none  TrackingMode=off  Kt=1  LimitOutput=on  UpperSaturationLimit=inf  LowerSaturationLimit=-inf  LinearizeAsGain=on  AntiWindupMode=clamping  Kb=1  POutMin=[]  POutMax=[]  IOutMin=[]  IOutMax=[]  DOutMin=[]  DOutMax=[]  NOutMin=[]  NOutMax=[]  SumOutMin=[]  SumOutMax=[]  SaturationOutMin=[]  SaturationOutMax=[]  PParamMin=[]  PParamMax=[]  IParamMin=[]  IParamMax=[]  DParamMin=[]  DParamMax=[]  NParamMin=[]  NParamMax=[]  KbParamMin=[]  KbParamMax=[]  KtParamMin=[]  KtParamMax=[]  KbOutMin=[]  KbOutMax=[]  KtOutMin=[]  KtOutMax=[]  IntegratorOutMin=[]  IntegratorOutMax=[]  FilterOutMin=[]  FilterOutMax=[]  SumI1OutMin=[]  SumI1OutMax=[]  SumI2OutMin=[]  SumI2OutMax=[]  SumI3OutMin=[]  SumI3OutMax=[]  SumI4OutMin=[]  SumI4OutMax=[]  SumDOutMin=[]  SumDOutMax=[]  DifferentiatorOutMin=[]  DifferentiatorOutMax=[]  FilterDiffOutCoefMin=[]  FilterDiffOutCoefMax=[]  ReciprocalOutMin=[]  ReciprocalOutMax=[]  SumDenOutMin=[]  SumDenOutMax=[]  SumNumOutMin=[]  SumNumOutMax=[]  DivideOutMin=[]  DivideOutMax=[]  IntegratorContinuousStateAttributes=''  IntegratorStateMustResolveToSignalObject=off  IntegratorRTWStateStorageClass=Auto  FilterContinuousStateAttributes=''  FilterStateMustResolveToSignalObject=off  FilterRTWStateStorageClass=Auto  ParallelPVariant=InternalParameters  IdealPVariant=Disabled  IVariant=InternalParameters  DVariant=Disabled  IntegratorVariant=Continuous  SatVariant=External  AWVariant=ContClampingParallel  PCopyVariant=Disabled  TRVariant=Disabled  FdbkBlocksVariant=Forward  IdealPFdbkVariant=Disabled  SatFdbkVariant=Disabled  DerivativeFilterVariant=Disabled  NVariant=Disabled  NCopyVariant=Disabled_SignalSpec  FilterICVariant=Disabled  IntegratorICVariant=InternalICs  ExternalResetVariant=Disabled  TRSumVariant=Passthrough  SumFdbkVariant=Disabled  SumVariant=Sum_PI
  PID Controller2 : simulink/Continuous/PID Controller  Controller=PI  Form=Parallel  TimeDomain=Continuous-time  SampleTime=-1  IntegratorMethod=Forward Euler  FilterMethod=Forward Euler  ControllerParametersSource=internal  P=w_P/w_LPF  I=w_P  D=0  UseFilter=on  N=100  TunerSelectOption=Transfer Function Based (PID Tuner App)  InitialConditionSource=internal  InitialConditionForIntegrator=-Q0/V0  InitialConditionForFilter=0  DifferentiatorICPrevScaledInput=0  ExternalReset=none  TrackingMode=off  Kt=1  LimitOutput=on  UpperSaturationLimit=Iqmax  LowerSaturationLimit=-Iqmax  LinearizeAsGain=on  AntiWindupMode=clamping  Kb=1  POutMin=[]  POutMax=[]  IOutMin=[]  IOutMax=[]  DOutMin=[]  DOutMax=[]  NOutMin=[]  NOutMax=[]  SumOutMin=[]  SumOutMax=[]  SaturationOutMin=[]  SaturationOutMax=[]  PParamMin=[]  PParamMax=[]  IParamMin=[]  IParamMax=[]  DParamMin=[]  DParamMax=[]  NParamMin=[]  NParamMax=[]  KbParamMin=[]  KbParamMax=[]  KtParamMin=[]  KtParamMax=[]  KbOutMin=[]  KbOutMax=[]  KtOutMin=[]  KtOutMax=[]  IntegratorOutMin=[]  IntegratorOutMax=[]  FilterOutMin=[]  FilterOutMax=[]  SumI1OutMin=[]  SumI1OutMax=[]  SumI2OutMin=[]  SumI2OutMax=[]  SumI3OutMin=[]  SumI3OutMax=[]  SumI4OutMin=[]  SumI4OutMax=[]  SumDOutMin=[]  SumDOutMax=[]  DifferentiatorOutMin=[]  DifferentiatorOutMax=[]  FilterDiffOutCoefMin=[]  FilterDiffOutCoefMax=[]  ReciprocalOutMin=[]  ReciprocalOutMax=[]  SumDenOutMin=[]  SumDenOutMax=[]  SumNumOutMin=[]  SumNumOutMax=[]  DivideOutMin=[]  DivideOutMax=[]  IntegratorContinuousStateAttributes=''  IntegratorStateMustResolveToSignalObject=off  IntegratorRTWStateStorageClass=Auto  FilterContinuousStateAttributes=''  FilterStateMustResolveToSignalObject=off  FilterRTWStateStorageClass=Auto  ParallelPVariant=InternalParameters  IdealPVariant=Disabled  IVariant=InternalParameters  DVariant=Disabled  IntegratorVariant=Continuous  SatVariant=Enabled  AWVariant=ContClampingParallel  PCopyVariant=Disabled  TRVariant=Disabled  FdbkBlocksVariant=Forward  IdealPFdbkVariant=Disabled  SatFdbkVariant=Disabled  DerivativeFilterVariant=Disabled  NVariant=Disabled  NCopyVariant=Disabled_SignalSpec  FilterICVariant=Disabled  IntegratorICVariant=InternalICs  ExternalResetVariant=Disabled  TRSumVariant=Passthrough  SumFdbkVariant=Disabled  SumVariant=Sum_PI
  PID Controller3 : simulink/Continuous/PID Controller  Controller=PI  Form=Parallel  TimeDomain=Continuous-time  SampleTime=-1  IntegratorMethod=Forward Euler  FilterMethod=Forward Euler  ControllerParametersSource=internal  P=w_V/w_LPF  I=w_V  D=0  UseFilter=on  N=100  TunerSelectOption=Transfer Function Based (PID Tuner App)  InitialConditionSource=internal  InitialConditionForIntegrator=-Q0/V0  InitialConditionForFilter=0  DifferentiatorICPrevScaledInput=0  ExternalReset=none  TrackingMode=off  Kt=1  LimitOutput=on  UpperSaturationLimit=Iqmax  LowerSaturationLimit=-Iqmax  LinearizeAsGain=on  AntiWindupMode=clamping  Kb=1  POutMin=[]  POutMax=[]  IOutMin=[]  IOutMax=[]  DOutMin=[]  DOutMax=[]  NOutMin=[]  NOutMax=[]  SumOutMin=[]  SumOutMax=[]  SaturationOutMin=[]  SaturationOutMax=[]  PParamMin=[]  PParamMax=[]  IParamMin=[]  IParamMax=[]  DParamMin=[]  DParamMax=[]  NParamMin=[]  NParamMax=[]  KbParamMin=[]  KbParamMax=[]  KtParamMin=[]  KtParamMax=[]  KbOutMin=[]  KbOutMax=[]  KtOutMin=[]  KtOutMax=[]  IntegratorOutMin=[]  IntegratorOutMax=[]  FilterOutMin=[]  FilterOutMax=[]  SumI1OutMin=[]  SumI1OutMax=[]  SumI2OutMin=[]  SumI2OutMax=[]  SumI3OutMin=[]  SumI3OutMax=[]  SumI4OutMin=[]  SumI4OutMax=[]  SumDOutMin=[]  SumDOutMax=[]  DifferentiatorOutMin=[]  DifferentiatorOutMax=[]  FilterDiffOutCoefMin=[]  FilterDiffOutCoefMax=[]  ReciprocalOutMin=[]  ReciprocalOutMax=[]  SumDenOutMin=[]  SumDenOutMax=[]  SumNumOutMin=[]  SumNumOutMax=[]  DivideOutMin=[]  DivideOutMax=[]  IntegratorContinuousStateAttributes=''  IntegratorStateMustResolveToSignalObject=off  IntegratorRTWStateStorageClass=Auto  FilterContinuousStateAttributes=''  FilterStateMustResolveToSignalObject=off  FilterRTWStateStorageClass=Auto  ParallelPVariant=InternalParameters  IdealPVariant=Disabled  IVariant=InternalParameters  DVariant=Disabled  IntegratorVariant=Continuous  SatVariant=Enabled  AWVariant=ContClampingParallel  PCopyVariant=Disabled  TRVariant=Disabled  FdbkBlocksVariant=Forward  IdealPFdbkVariant=Disabled  SatFdbkVariant=Disabled  DerivativeFilterVariant=Disabled  NVariant=Disabled  NCopyVariant=Disabled_SignalSpec  FilterICVariant=Disabled  IntegratorICVariant=InternalICs  ExternalResetVariant=Disabled  TRSumVariant=Passthrough  SumFdbkVariant=Disabled  SumVariant=Sum_PI
  PI_fw_init : Control_Lib/PI_fw_init  Kp=w_P/w_LPF  Ki=w_P
      settings: SourceProductName=VSC4SPS
  PI_fw_init1 : Control_Lib/PI_fw_init  Kp=w_P/w_LPF  Ki=w_P
      settings: SourceProductName=VSC4SPS
  PLL : Control_Lib/PLL  fb=fb  wn_PLL=wn_PLL  zeta_PLL=zeta_PLL  Theta0=Theta0
      settings: SourceProductName=VSC4SPS
  RMS derivation : Subsystem
  Saturation1 : Saturate  UpperLimit=Imax  LowerLimit=-Imax
  Saturation2 : Saturate  UpperLimit=Imax  LowerLimit=-Imax
  Scope1 : Scope  NumInputPorts=2
  Signal Conversion : SignalConversion  OverrideOpt=off
  Sqrt : Sqrt  SaturateOnIntegerOverflow=on
  Square : Math  Operator=square  SaturateOnIntegerOverflow=on
  Square1 : Math  Operator=square  SaturateOnIntegerOverflow=on
  Sum3 : Sum  Inputs=+-
  Sum4 : Sum  Inputs=+--
  Sum5 : Sum  Inputs=++-
  Sum6 : Sum  Inputs=+++
  Switch : Switch  Criteria=u2 > Threshold  Threshold=1.5
  abc2dq0_norm : Control_Lib/abc2dq0_norm  referenceAxisMode=Reference axis at 90 degrees behind phase_a  baseUpdateGain=1/sqrt(3)
      settings: SourceProductName=VSC4SPS
  dq02abc_norm : Control_Lib/dq02abc_norm  referenceAxisMode=Reference axis at 90 degrees behind phase_a  baseUpdateGain=sqrt(3)
      settings: SourceProductName=VSC4SPS
  norm1 : Subsystem
  norm2 : Subsystem
  vm_abc_ref_pu : Outport  VectorParamsAs1DForOutWhenUnconnected=off
  m : Outport  Port=2  VectorParamsAs1DForOutWhenUnconnected=off
  wires:
  [vg_abc_pu] -> Bus Creator2/3  "vg_abc_pu"
  Constant1/1 -> dq02abc_norm/2
  Mux/1 -> Inner Current Control/1(ig_dq_ref)
  Signal Conversion/1 -> m/1
  [P] -> Bus Creator/1  "P"
  [Q] -> Bus Creator/2  "Q"
  [w_PLL] -> Bus Creator/3  "f"
  dq02abc_norm/2 -> [vm_abc_ref_pu]  "vm_abc_pu"
  " pu P/Q computation"/2(Q) -> [Q]  "Q"
  [vm_dq] -> dq02abc_norm/1  "vm_dq"
  [w_PLL] -> Inner Current Control/3(w_PLL)
  Inner Current Control/1(vm_dq) -> [vm_dq]  "vm_dq"
  vg_abc_pu/1 -> [vg_abc_pu]
  " pu P/Q computation"/1(P) -> [P]  "P"
  ig_abc_pu/1 -> [ig_abc_pu]  "ig_abc_pu"
  abc2dq0_norm/2 -> [igdq]  "ig_dq"
  [CosSinTheta] -> CosSin_Delay/1
  [CosSinTheta] -> abc2dq0_norm/2
  Bus Creator2/1 -> [V]  "V"
  [V] -> Bus Creator/4  "V"
  Bus Creator/1 -> Signal Conversion/1
  Bus Creator1/1 -> [I]  "I"
  [I] -> Bus Creator/5  "I"
  LPF2/1(Out1) -> PI_fw_init/1, Add6/2
  P_set/1 -> [P_set]
  Add6/1 -> PID Controller2/1
  [P] -> LPF/1(In1)
  Add5/1 -> PID Controller1/1
  [Iqref_PI] -> Mux/2
  [Idref_PI] -> Mux/1
  [igdq] -> Inner Current Control/2(ig_dq)
  Saturation2/1 -> [Iqref]
  Sum4/1 -> Gain1/1
  [V_RMS] -> Sum4/2
  K_FRT/1 -> Saturation1/1
  Saturation1/1 -> Divide2/1
  Equal/1 -> Data Type Conversion/1
  Data Type Conversion/1 -> Divide2/2
  [vd] -> Equal/1
  Divide2/1 -> Add/1
  Constant12/1 -> Sum4/3
  Constant8/1 -> Sum4/1
  Constant9/1 -> Equal/2
  Constant4/1 -> Switch/2
  Add/1 -> Saturation2/1
  [Iqref_PI] -> Add/2
  Mux2/1 -> Inner Current Control/5(ig_dq_max)
  Constant5/1 -> Mux2/2
  [Idmax] -> Mux2/1
  [Q] -> LPF2/1(In1)
  Q_set/1 -> [Q_set]
  PID Controller2/1 -> Switch/1
  Add1/1 -> PID Controller3/1
  LPF1/1(Out1) -> Add1/2
  PID Controller3/1 -> Switch/3
  Square1/1 -> Sum3/2
  Sqrt/1 -> [Idmax]
  Sum3/1 -> Sqrt/1
  Constant3/1 -> Square/1
  Square/1 -> Sum3/1
  [Iqref] -> Square1/1
  Gain/1 -> PID Controller1/3
  Gain1/1 -> K_FRT/1
  Sum5/1 -> Mux3/1
  [vgdq] -> Gain3/1
  Demux2/2 -> Sum6/1
  Gain3/1 -> Demux2/1
  Constant2/1 -> Gain4/1
  norm1/1(Out1) -> [Vcomp]
  Divide1/1 -> Sum5/3
  Sum6/1 -> Mux3/2
  Mux3/1 -> norm1/1(In1)
  Divide/1 -> Sum6/3
  Divide5/1 -> Divide/2, Divide1/2
  Demux2/1 -> Sum5/1
  Divide3/1 -> Sum5/2
  Demux3/2 -> Divide1/1, Divide4/1
  Divide4/1 -> Sum6/2
  Demux3/1 -> Divide/1, Divide3/1
  PLL/1 -> [Theta_PLL]
  PLL/2 -> [CosSinTheta]
  PLL/3 -> [w_PLL]
  [w_PLL] -> Divide5/2
  Constant7/1 -> Gain5/1
  [Vpcc] -> LPF1/1(In1)
  Constant6/1 -> Add1/1
  [vg_abc_pu] -> PLL/1
  [vg_abc_pu] -> " pu P/Q computation"/1(v_abc_pu)
  [ig_abc_pu] -> " pu P/Q computation"/2(i_abc_pu)
  [ig_abc_pu] -> abc2dq0_norm/1
  [ig_abc_pu] -> Bus Creator1/1
  [igdq] -> Bus Creator1/2
  [vm_dq] -> Bus Creator2/2  "vm_dq"
  [vm_abc_ref_pu] -> vm_abc_ref_pu/1
  [vm_abc_ref_pu] -> Bus Creator2/1
  [vgdq] -> Inner Current Control/4(vg_dq)
  [P_set] -> PI_fw_init1/1, Add5/1
  [Q_set] -> PI_fw_init/2, Add6/1
  [igdq] -> Gain2/1
  Gain2/1 -> Demux3/1
  Gain5/1 -> Divide5/1
  Gain4/1 -> Divide4/2, Divide3/2
  [vgdq] -> norm2/1(In1)
  norm2/1(Out1) -> [Vpcc]
  PLL/4 -> Demux/1, [vgdq]
  Demux/1 -> [vd]
  Demux/2 -> [vq]
  LPF/1(Out1) -> PI_fw_init1/2, Add5/2
  [vgdq] -> RMS derivation/1(dq)
  RMS derivation/1(rms) -> Bus Creator2/4  "Vg_RMS"
  [Theta_PLL] -> Bus Creator3/1  "Theta"
  [CosSinTheta] -> Bus Creator3/2  "CosSinTheta"
  Bus Creator3/1 -> [Theta]  "Theta"
  [Theta] -> Bus Creator/6  "Theta"
  CosSin_Delay/1 -> dq02abc_norm/3
  LPF3/1(Out1) -> [V_RMS]
  [Vpcc] -> LPF3/1(In1)
  Constant/1 -> PID Controller1/2, Gain/1
  Constant10/1 -> PI_fw_init/5
  Constant11/1 -> PI_fw_init/4
  PI_fw_init/1 -> [Iqref_PI]
  Constant13/1 -> Scope1/2, PI_fw_init1/4
  Constant14/1 -> PI_fw_init1/5
  PI_fw_init1/1 -> [Idref_PI]
  [igdq] -> Scope1/1

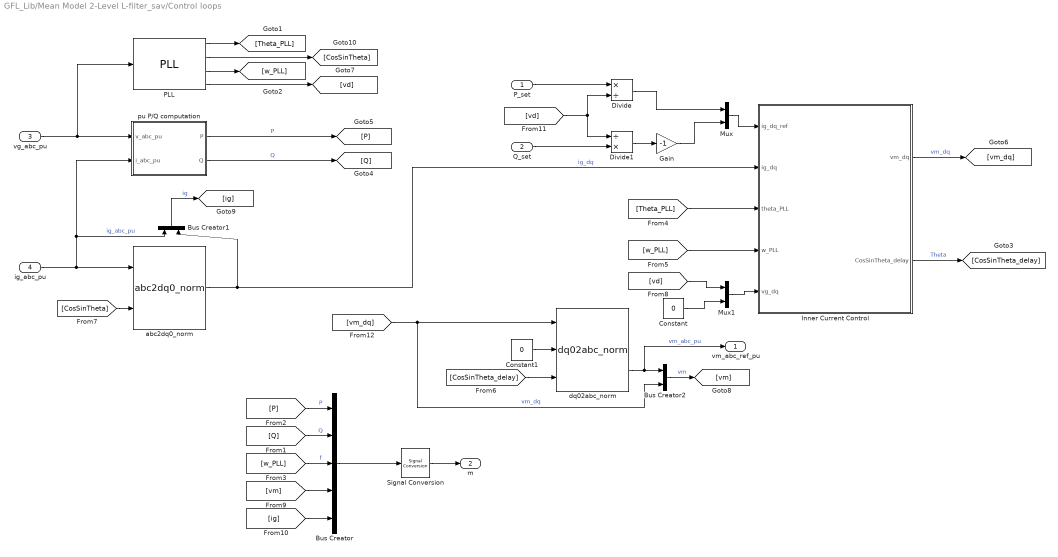
== system GFL_Lib/Mean Model 2-Level L-filter_sav/Control loops ==
  P_set : Inport
  Q_set : Inport  Port=2
  vg_abc_pu : Inport  Port=3
  ig_abc_pu : Inport  Port=4
  " pu P/Q computation" : Subsystem  DialogController=POWERSYS.PowerSysDialog
  Bus Creator : BusCreator  Inputs=5
  Bus Creator1 : BusCreator  Inputs=2
  Bus Creator2 : BusCreator  Inputs=2
  Constant : Constant  Value=0
  Constant1 : Constant  Value=0
  Divide : Product  Inputs=*/
  Divide1 : Product  Inputs=/*
  Gain : Gain  Gain=-1
  Inner Current Control : Subsystem
  Mux : Mux  Inputs=2
  Mux1 : Mux  Inputs=2
  PLL : Control_Lib/PLL  fb=fb  wn_PLL=wn_PLL  zeta_PLL=zeta_PLL  Theta0=Theta0
      settings: SourceProductName=VSC4SPS
  Signal Conversion : SignalConversion  OverrideOpt=off
  abc2dq0_norm : Control_Lib/abc2dq0_norm  referenceAxisMode=Reference axis at 90 degrees behind phase_a  baseUpdateGain=1/sqrt(3)
      settings: SourceProductName=VSC4SPS
  dq02abc_norm : Control_Lib/dq02abc_norm  referenceAxisMode=Reference axis at 90 degrees behind phase_a  baseUpdateGain=sqrt(3)
      settings: SourceProductName=VSC4SPS
  vm_abc_ref_pu : Outport  VectorParamsAs1DForOutWhenUnconnected=off
  m : Outport  Port=2  VectorParamsAs1DForOutWhenUnconnected=off
  wires:
  PLL/3 -> [w_PLL]
  PLL/1 -> [Theta_PLL]
  [ig] -> Bus Creator/5
  Bus Creator1/1 -> [ig]  "ig"
  Bus Creator/1 -> Signal Conversion/1
  [vm] -> Bus Creator/4
  Bus Creator2/1 -> [vm]  "vm"
  [CosSinTheta] -> abc2dq0_norm/2
  [CosSinTheta_delay] -> dq02abc_norm/3
  Inner Current Control/2(CosSinTheta_delay) -> [CosSinTheta_delay]  "Theta"
  abc2dq0_norm/2 -> Bus Creator1/2, Inner Current Control/2(ig_dq)  "ig_dq"
  ig_abc_pu/1 -> " pu P/Q computation"/2(i_abc_pu), Bus Creator1/1, abc2dq0_norm/1  "ig_abc_pu"
  " pu P/Q computation"/1(P) -> [P]  "P"
  vg_abc_pu/1 -> " pu P/Q computation"/1(v_abc_pu), PLL/1
  Inner Current Control/1(vm_dq) -> [vm_dq]  "vm_dq"
  [w_PLL] -> Inner Current Control/4(w_PLL)
  P_set/1 -> Divide/1
  [Theta_PLL] -> Inner Current Control/3(theta_PLL)
  [vm_dq] -> dq02abc_norm/1, Bus Creator2/2  "vm_dq"
  " pu P/Q computation"/2(Q) -> [Q]  "Q"
  Q_set/1 -> Divide1/2
  dq02abc_norm/2 -> vm_abc_ref_pu/1, Bus Creator2/1  "vm_abc_pu"
  [w_PLL] -> Bus Creator/3  "f"
  [Q] -> Bus Creator/2  "Q"
  [P] -> Bus Creator/1  "P"
  Signal Conversion/1 -> m/1
  PLL/4 -> [vd]
  [vd] -> Divide/2, Divide1/1
  Divide/1 -> Mux/1
  Divide1/1 -> Gain/1
  Mux/1 -> Inner Current Control/1(ig_dq_ref)
  [vd] -> Mux1/1
  Mux1/1 -> Inner Current Control/5(vg_dq)
  Constant/1 -> Mux1/2
  PLL/2 -> [CosSinTheta]
  Constant1/1 -> dq02abc_norm/2
  Gain/1 -> Mux/2

== system GFL_Lib/Mean Model 2-Level L-filter_sav/Mean_Model ==
  Uref : Inport
  Constant : Constant
  Memory : Memory
  NOT1 : Logic  Operator=NOT  IconShape=distinctive  AllPortsSameDT=off  OutDataTypeStr=boolean
  Terminator : Terminator
  Three-Phase Breaker1 : powerlib/Elements/Three-Phase Breaker  InitialState=closed  SwitchA=on  SwitchB=on  SwitchC=on  SwitchTimes="[4/60  10/60]"  External=on  BreakerResistance=0.001  SnubberResistance=1e6  SnubberCapacitance=inf  Measurements=None
  Three-Phase Breaker2 : powerlib/Elements/Three-Phase Breaker  InitialState=open  SwitchA=on  SwitchB=on  SwitchC=on  SwitchTimes="[4/60  10/60]"  External=on  BreakerResistance=0.001  SnubberResistance=1e6  SnubberCapacitance=inf  Measurements=None
  Three-Phase Source : powerlib/Electrical Sources/Three-Phase Source  InternalConnection=Yg  VoltagePhases=off  Voltage=Vvsc0*Un1  PhaseAngle=Theta_vsc0  Voltage_phases=[25e3 25e3 25e3]/sqrt(3)  PhaseAngles_phases=[0 -120 +120]  Frequency=fb  NonIdealSource=off  SpecifyImpedance=off  Resistance=0  Inductance=0  ShortCircuitLevel=100e6  BaseVoltage=VSC01_Un1  XRratio=7  BusType=swing  Pref=0.3  Qref=0  Prefabc=[10e3, 10e3, 10e3]  Qrefabc=[0, 0, 0]  Qmin=-Inf  Qmax=Inf
  Universal Bridge : powerlib/Power Electronics/Universal Bridge  Arms=3  SnubberResistance=1e5  SnubberCapacitance=inf  Device=Average-model based VSC  Ron=1e-3  Lon=0  ForwardVoltages="[  0  0  ]"  ForwardVoltage=0  GTOparameters=[ 10e-6 , 20e-6 ]  IGBTparameters=[ 1e-6 , 2e-6 ]  Measurements=None  Measurements_2=None  converterType=Rectifier
  Vdc : powerlib/Measurements/Voltage Measurement  PhasorSimulation=off  OutputType=Complex  PSBequivalent=0
  mp3 : Gain  Gain=2/Udcn
  PhA : PMIOPort  Side=Right
  PhB : PMIOPort  Port=2  Side=Right
  PhC : PMIOPort  Port=3  Side=Right
  Vdc+ : PMIOPort  Port=4  Side=Left
  Vdc- : PMIOPort  Port=5  Side=Left
  wires:
  NOT1/1 -> Three-Phase Breaker1/1
  Memory/1 -> NOT1/1, Three-Phase Breaker2/1
  mp3/1 -> Universal Bridge/1
  Uref/1 -> mp3/1
  Vdc/1 -> Terminator/1
  Constant/1 -> Memory/1
  connections:
  Three-Phase Breaker2/LConn1 -- Three-Phase Breaker1/LConn1 -- PhA/RConn1
  Three-Phase Breaker2/LConn2 -- Three-Phase Breaker1/LConn2 -- PhB/RConn1
  Three-Phase Breaker2/LConn3 -- Three-Phase Breaker1/LConn3 -- PhC/RConn1
  Three-Phase Breaker2/RConn1 -- Universal Bridge/LConn1
  Three-Phase Breaker2/RConn2 -- Universal Bridge/LConn2
  Three-Phase Breaker2/RConn3 -- Universal Bridge/LConn3
  Three-Phase Source/RConn1 -- Three-Phase Breaker1/RConn1
  Three-Phase Source/RConn2 -- Three-Phase Breaker1/RConn2
  Three-Phase Source/RConn3 -- Three-Phase Breaker1/RConn3
  Vdc/LConn1 -- Universal Bridge/RConn1 -- Vdc+/RConn1
  Vdc/LConn2 -- Universal Bridge/RConn2 -- Vdc-/RConn1
